simulink model "vipscenechange"  (R2015b)
settings: Solver=FixedStepDiscrete  StartTime=0.0  StopTime=inf  RelTol=1e-3
values from neighbouring files (symbols this model uses):
  sz = size(I)    [TextDetectionExample.m]    (also in videopatternmatching.m = get(0,'ScreenSize'); videostabilize.m = fileInfo.VideoSize)
undefined symbols (not defined in the file or in its folder): gray, M, N
libraries: vipmisc x4, simulink x3, visiontextngfix x2, visionsinks x2, visionstatistics x1, visionanalysis x1, dspvision x1
settings Model: FPTRunName=Active  ExtModeAutoUpdateStatusClock=off  Creator=The MathWorks, Inc.  LastModifiedBy=The MathWorks, Inc.
settings DataIOCC: LimitDataPoints=off  SaveFormat=Array  SaveOutput=off  SaveTime=off  SignalLoggingName=sigsOut
settings OptimizationCC: ExpressionDepthLimit=2147483647  LocalBlockOutputs=off  InitFltsAndDblsToZero=on  BufferReusableBoundary=off
settings DebuggingCC: SaveWithParameterizedLinksMsg=none  UnderspecifiedInitializationDetection=Classic  MergeDetectMultiDrivingBlocksExec=none  CheckExecutionContextPreStartOutputMsg=on  CheckExecutionContextRuntimeOutputMsg=on  SignalResolutionControl=TryResolveAllWithWarning  MultiTaskDSMMsg=warning  MultiTaskCondExecSysMsg=none  FcnCallInpInsideContextMsg=UseLocalSettings  BusObjectLabelMismatch=none  StateNameClashWarn=warning  StrictBusMsg=None
settings HardwareCC: ProdBitPerPointer=32  ProdLargestAtomicFloat=None  ProdIntDivRoundTo=Undefined  ProdEndianess=Unspecified  ProdWordSize=32  ProdHWDeviceType=32-bit Generic  TargetBitPerLong=64  TargetBitPerPointer=64  TargetLongLongMode=on  TargetIntDivRoundTo=Zero  TargetEndianess=LittleEndian  TargetWordSize=64  TargetHWDeviceType=Generic->MATLAB Host Computer  ProdEqTarget=off
settings GRTTargetCC: TargetFcnLib=ansi_tfl_tmw.mat  GeneratePreprocessorConditionals=Disable all  CombineOutputUpdateFcns=off  GRTInterface=on
settings ConfigComp: CovModelRefEnable=Off

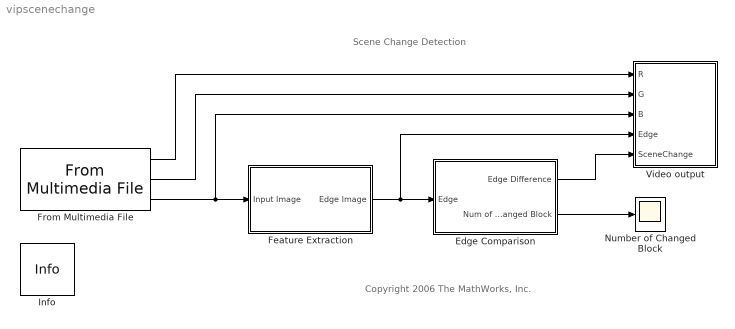
== system vipscenechange ==
  note: Scene Change Detection
  note: Copyright 2006 The MathWorks, Inc.
  Edge Comparison : Subsystem
  Feature Extraction : Subsystem
  From Multimedia File : dspvision/From Multimedia File  inputFilename=vipscenevideoclip.avi  loop=on  numPlays=inf  outputStreams=Video and audio  videoDataType=single  audioDataType=int16  inheritSampleTime=on  userDefinedSampleTime=1/30  noAudioOutput=off  isIntensityVideo=off  fourcc=RGB  colorVideoFormat=Separate color signals  outputEOF=off  dataOrg=Column-major  audioFrameSize=1024  computeAudioFrameSize=off  outSamplingMode=Frame based
  Info : vipmisc/Info  SystemSampleTime=-1
  Number of Changed Block : Scope
  Video output : Subsystem
  wires:
  Feature Extraction/1(Edge Image) -> Video output/4(Edge), Edge Comparison/1(Edge)
  From Multimedia File/1 -> Video output/1(R)
  Edge Comparison/2(Num of Changed Block) -> Number of Changed Block/1
  From Multimedia File/2 -> Video output/2(G)
  From Multimedia File/3 -> Feature Extraction/1(Input Image), Video output/3(B)
  Edge Comparison/1(Edge Difference) -> Video output/5(SceneChange)

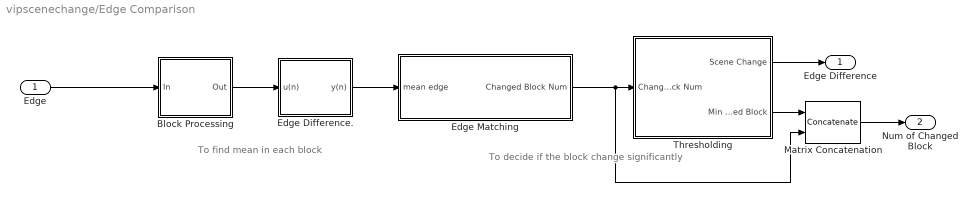
== system vipscenechange/Edge Comparison ==
  note: To find mean in each block
  note: To decide if the block change significantly
  Edge : Inport
  Block Processing : Subsystem  DialogController=vipDDGCreate  TreatAsAtomicUnit=on  mask(Block Processing){NumI=1, ParamPort=off, NumO=1, Blocksize={[32 32]}, Overlapsize={[0 0]}, Traverse=Row-wise}
      mask prompts: NumI "Number of inputs:"; ParamPort "Add port to supply subsystem parameters"; NumO "Number of outputs:"; Blocksize "Block size:"; Overlapsize "Overlap size:"; Traverse "Order of traversing:"
      mask help:
      | Repeats a user-specified operation on submatrices of the input matrix.
      |
      | This block extracts submatrices of a user-specified size from the input matrix. It sends each submatrix to a subsystem for processing, and then reassembles each subsystem output into the output matrix.
      |
      | Use the Block size and Overlap parameters to specify the size and overlap of each submatrix in cell array format.
      mask init:
      | errmsg = vipblkblockproc(gcbh, NumI, NumO, Blocksize, Overlapsize, Traverse, ParamPort);
      | error(errmsg);
      settings: CopyFcn=set_param(gcb,'LinkStatus','none');
      mask Help: eval('helpview(fullfile(docroot,''toolbox'',''vision'',''vision.map''),''vipblockprocessing'')');
      mask TypeOptions Traverse: Row-wise | Column-wise
      mask Display:
      | disp('Block\n Processing');
      | 
      | if ((NumI == 1) && ParamPort)
      |     port_label('input', 1, 'I');
      | end
      | 
      | if (NumI > 1)
      |     for (i = 1:NumI)
      |         port_label('input', i, ['I' int2str(i)]);
      |     end
      | end
      | 
      | if (ParamPort)
      |     port_label('input', NumI+1, 'P');
      | end
  Edge Difference. : Subsystem
  Edge Matching : Subsystem
  Matrix Concatenation : Concatenate  Mode=Multidimensional array  ConcatenateDimension=2
  Thresholding : Subsystem
  Edge Difference : Outport
  Num of Changed Block : Outport  Port=2
  wires:
  Edge Matching/1(Changed Block Num) -> Thresholding/1(Changed Block Num), Matrix Concatenation/2
  Edge/1 -> Block Processing/1(In)
  Thresholding/1(Scene Change) -> Edge Difference/1
  Block Processing/1(Out) -> Edge Difference./1(u(n))
  Edge Difference./1(y(n)) -> Edge Matching/1(mean edge)
  Thresholding/2(Min Num of Changed Block) -> Matrix Concatenation/1
  Matrix Concatenation/1 -> Num of Changed Block/1

== system vipscenechange/Feature Extraction ==
  Input Image : Inport
  Data Type Conversion : DataTypeConversion  OutDataTypeStr=single  SaturateOnIntegerOverflow=on  RndMeth=Zero
  Edge Detection1 : visionanalysis/Edge Detection  method=Sobel  outputType=Binary image  userDefinedThreshold=off  thresholdSource=Specify via dialog  threshold=15/256  thresholdTuning=single(3)  edgeThinning=on  threshold_canny=[0.25 0.60]  autoPercent=70  sigma=1  roundingMode=Floor  overflowMode=off
  Edge Image : Outport
  wires:
  Edge Detection1/1 -> Data Type Conversion/1
  Input Image/1 -> Edge Detection1/1
  Data Type Conversion/1 -> Edge Image/1

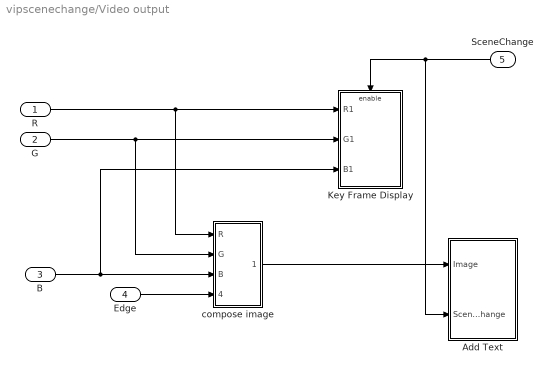
== system vipscenechange/Video output ==
  R : Inport
  G : Inport  Port=2
  B : Inport  Port=3
  Edge : Inport  Port=4
  SceneChange : Inport  Port=5
  Add Text : Subsystem
  Key Frame Display : Subsystem
  compose image : Subsystem
  wires:
  R/1 -> compose image/1(R), Key Frame Display/1(R1)
  B/1 -> compose image/3(B), Key Frame Display/3(B1)
  SceneChange/1 -> Key Frame Display/Enable, Add Text/2(Scene Change)
  G/1 -> compose image/2(G), Key Frame Display/2(G1)
  Edge/1 -> compose image/4(edge)
  compose image/1(Image) -> Add Text/1(Image)

== system vipscenechange/Edge Comparison/Block Processing ==
  In : Inport
  Block iterator : Subsystem
      settings: CopyFcn=set_param(gcb,'ReferenceBlock','');
  Iteration count : vipmisc/Iteration count  NumI=NumI  blksize=Blocksize  ovlpsize=Overlapsize
  Out : Outport
  wires:
  Iteration count/1 -> Block iterator/1(iter)
  In/1 -> Iteration count/1, Block iterator/2(In1)
  Block iterator/1(Out) -> Out/1

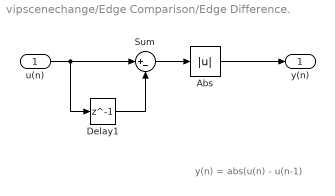
== system vipscenechange/Edge Comparison/Edge Difference. ==
  note: y(n) = abs(u(n) - u(n-1)
  u(n) : Inport
  Abs : Abs  SaturateOnIntegerOverflow=on
  Delay1 : Delay  DelayLength=1  InitialCondition=0
  Sum : Sum  Inputs=|+-  SaturateOnIntegerOverflow=on  InputSameDT=on  OutDataTypeStr=Inherit: Same as first input
  y(n) : Outport
  wires:
  Abs/1 -> y(n)/1
  Sum/1 -> Abs/1
  Delay1/1 -> Sum/2
  u(n)/1 -> Sum/1, Delay1/1

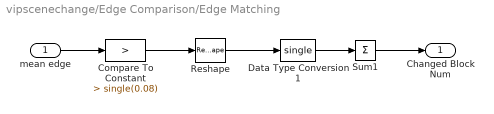
== system vipscenechange/Edge Comparison/Edge Matching ==
  mean edge : Inport
  Compare To Constant : simulink/Logic and Bit Operations/Compare To Constant  relop=>  const=single(0.08)  OutDataTypeStr=boolean  ZeroCross=off
  Data Type Conversion1 : DataTypeConversion  OutDataTypeStr=single  SaturateOnIntegerOverflow=on  RndMeth=Zero
  Reshape : Reshape  OutputDimensionality=Column vector (2-D)
  Sum1 : Sum  Inputs=+  SaturateOnIntegerOverflow=on  InputSameDT=on  OutDataTypeStr=Inherit: Same as first input
  Changed Block Num : Outport
  wires:
  Reshape/1 -> Data Type Conversion1/1
  Sum1/1 -> Changed Block Num/1
  Compare To Constant/1 -> Reshape/1
  mean edge/1 -> Compare To Constant/1
  Data Type Conversion1/1 -> Sum1/1

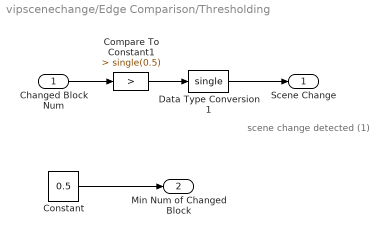
== system vipscenechange/Edge Comparison/Thresholding ==
  note: scene change detected (1)
  Changed Block Num : Inport
  Compare To Constant1 : simulink/Logic and Bit Operations/Compare To Constant  relop=>  const=single(0.5)  OutDataTypeStr=boolean  ZeroCross=off
  Constant : Constant  Value=0.5  OutDataTypeStr=single
  Data Type Conversion1 : DataTypeConversion  OutDataTypeStr=single  SaturateOnIntegerOverflow=on  RndMeth=Zero
  Scene Change : Outport
  Min Num of Changed Block : Outport  Port=2
  wires:
  Changed Block Num/1 -> Compare To Constant1/1
  Data Type Conversion1/1 -> Scene Change/1
  Constant/1 -> Min Num of Changed Block/1
  Compare To Constant1/1 -> Data Type Conversion1/1

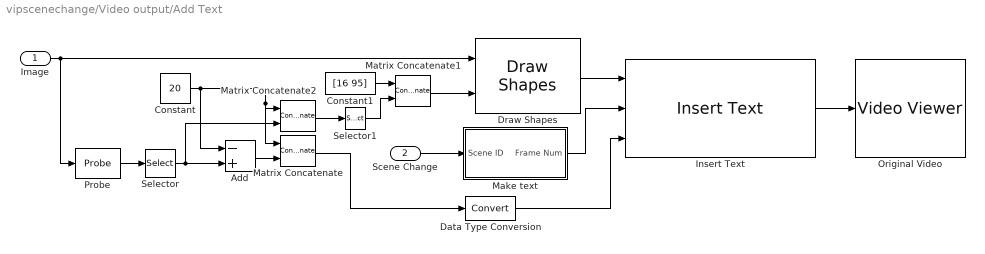
== system vipscenechange/Video output/Add Text ==
  Image : Inport
  Scene Change : Inport  Port=2
  Add : Sum  Inputs=-+
  Constant : Constant  Value=20
  Constant1 : Constant  Value=[16 95]  VectorParams1D=off
  Data Type Conversion : DataTypeConversion
  Draw Shapes : visiontextngfix/Draw Shapes  shape=Rectangles  fill=on  lineWidth=1  fillClrSource=Specify via dialog  display=Black  intensity=200  color=[0 50 0]  opacity=0.75  viewport=Entire image  antialiasing=off  inType=Obsolete  imagePorts=One multidimensional signal  prodOutputMode=Binary point scaling  prodOutputWordLength=32  prodOutputFracLength=14  memoryMode=Specify word length  memoryWordLength=16  memoryFracLength=14  roundingMode=Floor  overflowMode=off
  Insert Text : visiontextngfix/Insert Text  inputType=Obsolete  theText="'Frame%4d  Shot%2d'"  getTextLocFrom=Input port  textLoc=[100 20]  getTextColorFrom=Specify via dialog  textColor=[0 1 0]  getTextIntensityFrom=Specify via dialog  textIntensity=45/256  getTextOpacityFrom=Specify via dialog  textOpacity=1.0  dummyVar2=0  dummyVar3=0  dummyVar4=0  imagePorts=One multidimensional signal  isInputTransposed=off  fontFace=LucidaSansRegular  dummyVar1=0  blockFontSize=12  antiAliased=on
  Make text : Subsystem
  Matrix Concatenate : Concatenate  Mode=Multidimensional array  ConcatenateDimension=2
  Matrix Concatenate1 : Concatenate  Mode=Multidimensional array  ConcatenateDimension=2
  Matrix Concatenate2 : Concatenate  Mode=Multidimensional array  ConcatenateDimension=2
  Original Video : visionsinks/Video Viewer  inputType=Obsolete7b  imagePorts=One multidimensional signal  useColorMap=off  colormapValue=gray(256)  specRange=off  minInputVal=0  maxInputVal=255  FigPos=[528 274 320 145]  AxisZoom=on  trueSizedOnce=on  OpenAtMdlStart=on  DefaultConfigurationName=vipscopes.VideoViewerScopeCfg
  Probe : Probe  ProbeWidth=off  ProbeSampleTime=off  ProbeComplexSignal=off  ProbeSignalDimensions=on
  Selector : Selector  InputPortWidth=3  IndexOptions=Index vector (dialog)  Indices=1  OutputSizes=1
  Selector1 : Selector  NumberOfDimensions=2  InputPortWidth=3  IndexOptions=Select all,Index vector (dialog)  Indices=[1 3],[2 1]  OutputSizes=1,1
  wires:
  Scene Change/1 -> Make text/1(Scene ID)
  Image/1 -> Probe/1, Draw Shapes/1
  Insert Text/1 -> Original Video/1
  Make text/1(Frame Num) -> Insert Text/2
  Probe/1 -> Selector/1
  Data Type Conversion/1 -> Insert Text/3
  Draw Shapes/1 -> Insert Text/1
  Matrix Concatenate1/1 -> Draw Shapes/2
  Selector/1 -> Add/2, Matrix Concatenate2/2
  Constant/1 -> Add/1, Matrix Concatenate/1, Matrix Concatenate2/1
  Constant1/1 -> Matrix Concatenate1/1
  Add/1 -> Matrix Concatenate/2
  Matrix Concatenate/1 -> Data Type Conversion/1
  Matrix Concatenate2/1 -> Selector1/1
  Selector1/1 -> Matrix Concatenate1/2

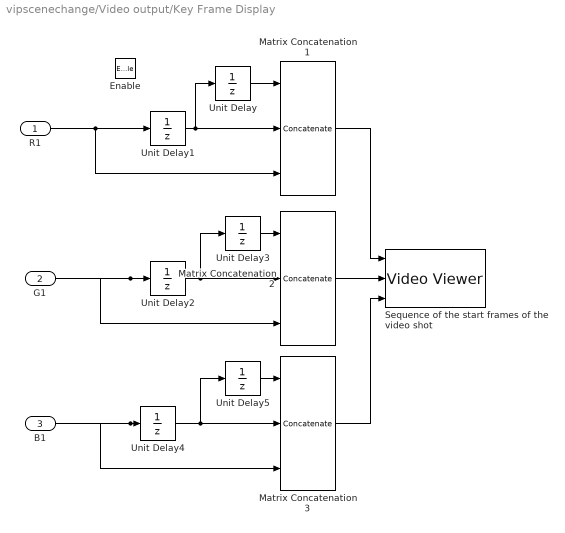
== system vipscenechange/Video output/Key Frame Display ==
  R1 : Inport
  G1 : Inport  Port=2
  B1 : Inport  Port=3
  Enable : EnablePort  PropagateVarSize=During execution
  Matrix Concatenation1 : Concatenate  NumInputs=3  Mode=Multidimensional array  ConcatenateDimension=2
  Matrix Concatenation2 : Concatenate  NumInputs=3  Mode=Multidimensional array  ConcatenateDimension=2
  Matrix Concatenation3 : Concatenate  NumInputs=3  Mode=Multidimensional array  ConcatenateDimension=2
  Sequence of the start frames of the video shot : visionsinks/Video Viewer  inputType=Obsolete7b  imagePorts=Separate color signals  useColorMap=off  colormapValue=gray(256)  specRange=off  minInputVal=0  maxInputVal=255  FigPos=[24 273 480 144]  AxisZoom=on  trueSizedOnce=on  OpenAtMdlStart=on  DefaultConfigurationName=vipscopes.VideoViewerScopeCfg
  Unit Delay{,1..5} (6 alike) : UnitDelay  SampleTime=-1
  wires:
  Matrix Concatenation3/1 -> Sequence of the start frames of the video shot/3
  B1/1 -> Matrix Concatenation3/3, Unit Delay4/1
  Unit Delay5/1 -> Matrix Concatenation3/1
  Unit Delay4/1 -> Matrix Concatenation3/2, Unit Delay5/1
  Matrix Concatenation2/1 -> Sequence of the start frames of the video shot/2
  G1/1 -> Matrix Concatenation2/3, Unit Delay2/1
  Unit Delay3/1 -> Matrix Concatenation2/1
  Unit Delay2/1 -> Matrix Concatenation2/2, Unit Delay3/1
  Matrix Concatenation1/1 -> Sequence of the start frames of the video shot/1
  R1/1 -> Matrix Concatenation1/3, Unit Delay1/1
  Unit Delay/1 -> Matrix Concatenation1/1
  Unit Delay1/1 -> Matrix Concatenation1/2, Unit Delay/1

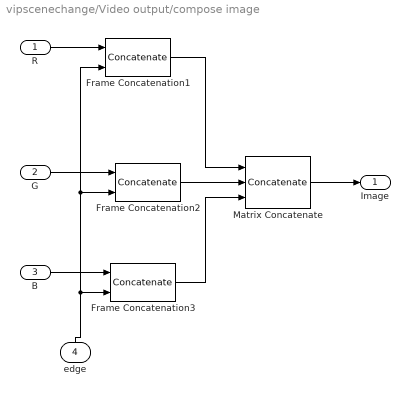
== system vipscenechange/Video output/compose image ==
  R : Inport
  G : Inport  Port=2
  B : Inport  Port=3
  edge : Inport  Port=4
  Frame Concatenation1 : Concatenate  Mode=Multidimensional array  ConcatenateDimension=2
  Frame Concatenation2 : Concatenate  Mode=Multidimensional array  ConcatenateDimension=2
  Frame Concatenation3 : Concatenate  Mode=Multidimensional array  ConcatenateDimension=2
  Matrix Concatenate : Concatenate  NumInputs=3  Mode=Multidimensional array  ConcatenateDimension=3
  Image : Outport
  wires:
  R/1 -> Frame Concatenation1/1
  G/1 -> Frame Concatenation2/1
  Frame Concatenation1/1 -> Matrix Concatenate/1
  edge/1 -> Frame Concatenation2/2, Frame Concatenation1/2, Frame Concatenation3/2
  B/1 -> Frame Concatenation3/1
  Frame Concatenation3/1 -> Matrix Concatenate/3
  Matrix Concatenate/1 -> Image/1
  Frame Concatenation2/1 -> Matrix Concatenate/2

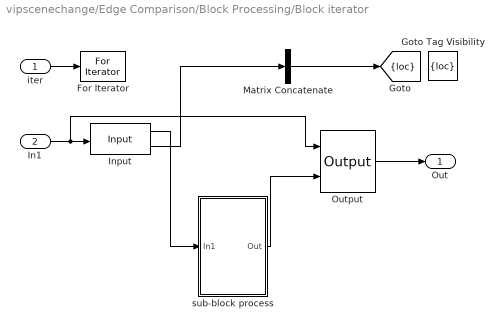
== system vipscenechange/Edge Comparison/Block Processing/Block iterator ==
  iter : Inport
  In1 : Inport  Port=2
  For Iterator : ForIterator  IterationSource=external  IterationLimit=(sz(1)/M)*(sz(2)/N)  ShowIterationPort=off  IndexMode=Zero-based  IterationVariableDataType=double
  Goto Tag Visibility : GotoTagVisibility  GotoTag=loc
  Input : vipmisc/Input  Blocksize=Blocksize{1}  Overlapsize=Overlapsize{1}  tverse=Row-wise
  Matrix Concatenate : Concatenate  NumInputs=1  Mode=Multidimensional array  ConcatenateDimension=2
  Output : vipmisc/Output  Blocksize=Blocksize{1}  Overlapsize=Overlapsize{1}  tverse=Row-wise
  sub-block process : Subsystem
  Out : Outport
  tag scope: loc=scoped
  wires:
  Matrix Concatenate/1 -> [loc]
  Input/2 -> Matrix Concatenate/1
  Input/1 -> sub-block process/1(In1)
  iter/1 -> For Iterator/1
  In1/1 -> Input/1, Output/1
  Output/1 -> Out/1
  sub-block process/1(Out) -> Output/2

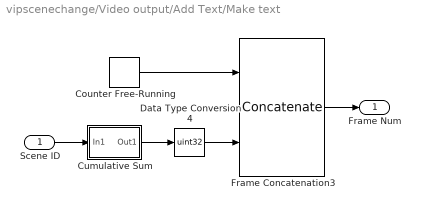
== system vipscenechange/Video output/Add Text/Make text ==
  Scene ID : Inport
  Counter Free-Running : simulink/Sources/Counter Free-Running  NumBits=32  tsamp=-1
  Cumulative Sum : Subsystem
  Data Type Conversion4 : DataTypeConversion  OutDataTypeStr=uint32  RndMeth=Zero
  Frame Concatenation3 : Concatenate  Mode=Multidimensional array  ConcatenateDimension=2
  Frame Num : Outport
  wires:
  Counter Free-Running/1 -> Frame Concatenation3/1
  Cumulative Sum/1(Out1) -> Data Type Conversion4/1
  Data Type Conversion4/1 -> Frame Concatenation3/2
  Scene ID/1 -> Cumulative Sum/1(In1)
  Frame Concatenation3/1 -> Frame Num/1

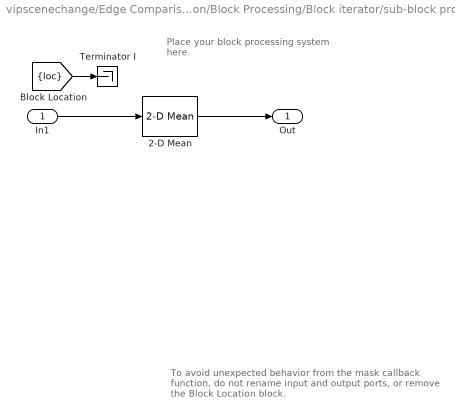
== system vipscenechange/Edge Comparison/Block Processing/Block iterator/sub-block process ==
  note: To avoid unexpected behavior from the mask
      | callback function, do not rename input and output ports,
      | or remove the Block Location block.
  note: Place your block
      | processing system here.
  In1 : Inport
  2-D Mean : visionstatistics/2-D Mean  run=off  reset_popup=None  directionMode=Entire input  dimension=1  treatSBRowAsCol=on  roiEnable=off  roiType=Rectangles  roiPortion=Entire ROI  roiOutput=Individual statistics for each ROI  roiFlag=off  outputDataTypeStr=Inherit: Same as accumulator  outputLastDataTypeStr=Inherit: Same as accumulator  outputMin=[]  outputMax=[]  accumMode=Binary point scaling  accumWordLength=32  accumFracLength=0  accumDataTypeStr=fixdt([],32,0)  accumLastDataTypeStr=fixdt([],32,0)  roundingMode=Floor  overflowMode=off
  Terminator I : Terminator
  Out : Outport
  wires:
  [loc] -> Terminator I/1
  In1/1 -> 2-D Mean/1
  2-D Mean/1 -> Out/1

== system vipscenechange/Video output/Add Text/Make text/Cumulative Sum ==
  In1 : Inport
  Sum of Elements : Sum
  Unit Delay : UnitDelay  SampleTime=-1
  Out1 : Outport
  wires:
  In1/1 -> Sum of Elements/1
  Unit Delay/1 -> Sum of Elements/2
  Sum of Elements/1 -> Out1/1, Unit Delay/1
